simulink model "SpeedControl"  (Simulink 7.7)
settings: Solver=ode45  StartTime=0.0  StopTime=8  FixedStep=1e-6  RelTol=1e-3
InitFcn:
  | load SpeedControl.mat
values from neighbouring files (symbols this model uses):
  detaGND = 1.6    [SpeedControl.mat]
  Ts = 0.01    [SpeedControl.mat]
  WnGND = 1.5    [SpeedControl.mat]
libraries: simulink x1
settings Model: Creator=Administrator  LastModifiedBy=chenx

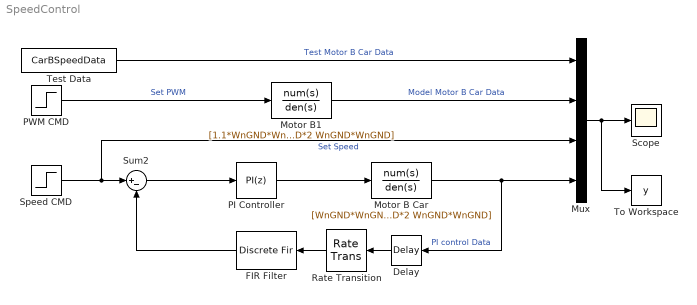
== system SpeedControl ==
  Delay : TransportDelay  DelayTime=0.005
  FIR Filter : DiscreteFir  NumCoeffs=[1 1 1 1]/4
  Motor B Car : TransferFcn  Numerator=[WnGND*WnGND]  Denominator=[1 WnGND*detaGND*2 WnGND*WnGND]
  Motor B1 : TransferFcn  Numerator=[1.1*WnGND*WnGND]  Denominator=[1.0 WnGND*detaGND*2 WnGND*WnGND]
  Mux : Mux
  PI Controller : simulink/Continuous/PID Controller  SystemSampleTime=-1  Controller=PI  TimeDomain=Discrete-time  SampleTime=Ts  IntegratorMethod=Forward Euler  FilterMethod=Forward Euler  Form=Parallel  P=4  I=2.5  D=0.0364210490711884  N=189.887708441779  InitialConditionSource=internal  InitialConditionForIntegrator=0  InitialConditionForFilter=0  ExternalReset=none  LimitOutput=on  UpperSaturationLimit=1000  LowerSaturationLimit=-1000  LinearizeAsGain=off  AntiWindupMode=clamping  Kb=1  TrackingMode=off  Kt=1  PParamMin=[]  PParamMax=[]  IParamMin=[]  IParamMax=[]  DParamMin=[]  DParamMax=[]  NParamMin=[]  NParamMax=[]  KbParamMin=[]  KbParamMax=[]  KtParamMin=[]  KtParamMax=[]  POutMin=[]  POutMax=[]  IOutMin=[]  IOutMax=[]  DOutMin=[]  DOutMax=[]  NOutMin=[]  NOutMax=[]  KbOutMin=[]  KbOutMax=[]  KtOutMin=[]  KtOutMax=[]  IntegratorOutMin=[]  IntegratorOutMax=[]  FilterOutMin=[]  FilterOutMax=[]  SumOutMin=[]  SumOutMax=[]  SumI1OutMin=[]  SumI1OutMax=[]  SumI2OutMin=[]  SumI2OutMax=[]  SumI3OutMin=[]  SumI3OutMax=[]  SumDOutMin=[]  SumDOutMax=[]  SaturationOutMin=[]  SaturationOutMax=[]  IntegratorContinuousStateAttributes=''  IntegratorStateMustResolveToSignalObject=off  IntegratorRTWStateStorageClass=Auto  FilterContinuousStateAttributes=''  FilterStateMustResolveToSignalObject=off  FilterRTWStateStorageClass=Auto
  PWM CMD : Step  Time=0  After=250  SampleTime=Ts
  Rate Transition : RateTransition  OutPortSampleTime=Ts
  Scope : Scope
      settings: YMin=0  YMax=275
  Speed CMD : Step  Time=0  After=260  SampleTime=Ts
  Sum2 : Sum  Inputs=|+-  SampleTime=Ts
  Test Data : FromWorkspace  VariableName=CarBSpeedData  SampleTime=0.01
  To Workspace : ToWorkspace  VariableName=y  SampleTime=-1  SaveFormat=Array
  wires:
  Mux/1 -> Scope/1, To Workspace/1
  Sum2/1 -> PI Controller/1
  Rate Transition/1 -> FIR Filter/1
  FIR Filter/1 -> Sum2/2
  Delay/1 -> Rate Transition/1
  Motor B Car/1 -> Delay/1, Mux/4  "PI control Data"
  Motor B1/1 -> Mux/2  "Model Motor B Car Data"
  Test Data/1 -> Mux/1  "Test Motor B Car Data"
  PI Controller/1 -> Motor B Car/1
  PWM CMD/1 -> Motor B1/1  "Set PWM"
  Speed CMD/1 -> Sum2/1, Mux/3  "Set Speed"
